simulink model "IP_order2_simscape_all_pre"  (R2019b)
settings: Solver=FixedStepAuto  StartTime=0.0  StopTime=15  FixedStep=1e-3  RelTol=1e-3
values from neighbouring files (symbols this model uses):
  K = K_lqr    [main_order2.m]
  K_lqr = lqr(A,B,Q,R)    [main_order2.m]
settings Model: Creator=cc  LastModifiedBy=zyinx
settings DebuggingCC: SFMachineParentedDataDiag=error

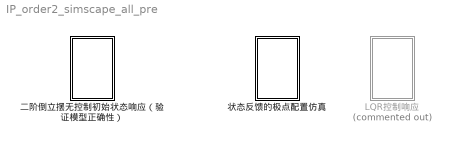
== system IP_order2_simscape_all_pre ==
  LQR控制响应 : Subsystem  Commented=on
  二阶倒立摆无控制初始状态响应（验证模型正确性） : Subsystem
  状态反馈的极点配置仿真 : Subsystem

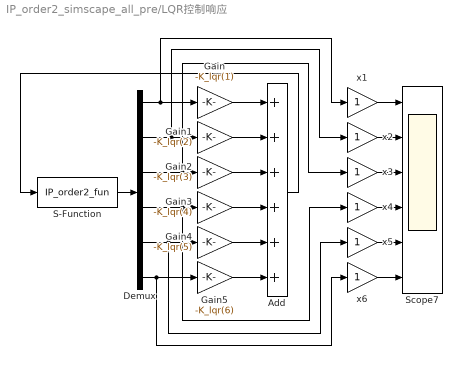
== system IP_order2_simscape_all_pre/LQR控制响应 ==
  Add : Sum  Inputs=++++++
  Demux : Demux  Outputs=6
  Gain : Gain  Gain=-K_lqr(1)
  Gain1 : Gain  Gain=-K_lqr(2)
  Gain2 : Gain  Gain=-K_lqr(3)
  Gain3 : Gain  Gain=-K_lqr(4)
  Gain4 : Gain  Gain=-K_lqr(5)
  Gain5 : Gain  Gain=-K_lqr(6)
  S-Function : S-Function  FunctionName=IP_order2_fun  Parameters=0; 0; 0; 0; 0; 5/180*pi  SFunctionDeploymentMode=off  EnableBusSupport=off
  Scope7 : Scope  NumInputPorts=6
  x{1..6} (6 alike) : Gain
  wires:
  S-Function/1 -> Demux/1
  Demux/1 -> x1/1, Gain/1
  Demux/2 -> Gain1/1, x2/1
  Demux/3 -> x3/1, Gain2/1
  Demux/4 -> x4/1, Gain3/1
  Demux/5 -> x5/1, Gain4/1
  Demux/6 -> x6/1, Gain5/1
  Gain/1 -> Add/1
  Gain1/1 -> Add/2
  Gain2/1 -> Add/3
  Gain3/1 -> Add/4
  Gain4/1 -> Add/5
  Gain5/1 -> Add/6
  Add/1 -> S-Function/1
  x1/1 -> Scope7/1
  x2/1 -> Scope7/2
  x3/1 -> Scope7/3
  x4/1 -> Scope7/4
  x5/1 -> Scope7/5
  x6/1 -> Scope7/6

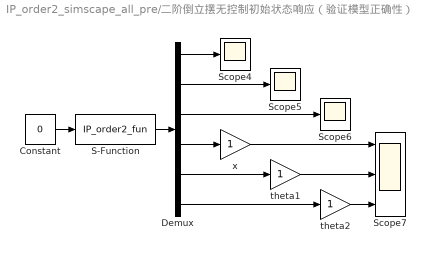
== system IP_order2_simscape_all_pre/二阶倒立摆无控制初始状态响应（验证模型正确性） ==
  Constant : Constant  Value=0
  Demux : Demux  Outputs=6
  S-Function : S-Function  FunctionName=IP_order2_fun  Parameters=0; 0; 0; 0; pi; 5/6*pi  SFunctionDeploymentMode=off  EnableBusSupport=off
  Scope4 : Scope
  Scope5 : Scope
  Scope6 : Scope
  Scope7 : Scope  NumInputPorts=3
  theta1 : Gain
  theta2 : Gain
  x : Gain
  wires:
  x/1 -> Scope7/1
  Demux/2 -> Scope5/1
  Constant/1 -> S-Function/1
  theta2/1 -> Scope7/3
  Demux/5 -> theta1/1
  theta1/1 -> Scope7/2
  Demux/6 -> theta2/1
  Demux/3 -> Scope6/1
  Demux/4 -> x/1
  S-Function/1 -> Demux/1
  Demux/1 -> Scope4/1

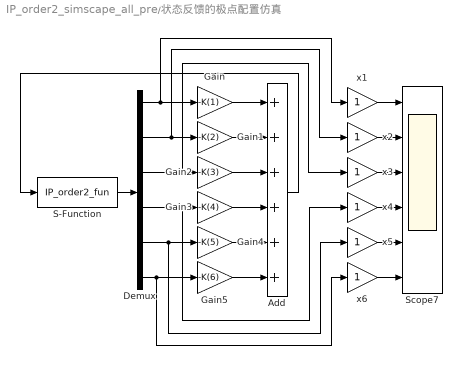
== system IP_order2_simscape_all_pre/状态反馈的极点配置仿真 ==
  Add : Sum  Inputs=++++++
  Demux : Demux  Outputs=6
  Gain : Gain  Gain=-K(1)
  Gain1 : Gain  Gain=-K(2)
  Gain2 : Gain  Gain=-K(3)
  Gain3 : Gain  Gain=-K(4)
  Gain4 : Gain  Gain=-K(5)
  Gain5 : Gain  Gain=-K(6)
  S-Function : S-Function  FunctionName=IP_order2_fun  Parameters=0; 0; 0; 0; 0; 5/180*pi  SFunctionDeploymentMode=off  EnableBusSupport=off
  Scope7 : Scope  NumInputPorts=6
  x{1..6} (6 alike) : Gain
  wires:
  S-Function/1 -> Demux/1
  Demux/1 -> x1/1, Gain/1
  Demux/2 -> Gain1/1, x2/1
  Demux/3 -> x3/1, Gain2/1
  Demux/4 -> x4/1, Gain3/1
  Demux/5 -> x5/1, Gain4/1
  Demux/6 -> x6/1, Gain5/1
  Gain/1 -> Add/1
  Gain1/1 -> Add/2
  Gain2/1 -> Add/3
  Gain3/1 -> Add/4
  Gain4/1 -> Add/5
  Gain5/1 -> Add/6
  Add/1 -> S-Function/1
  x1/1 -> Scope7/1
  x2/1 -> Scope7/2
  x3/1 -> Scope7/3
  x4/1 -> Scope7/4
  x5/1 -> Scope7/5
  x6/1 -> Scope7/6
